simulink model "SF015A_WhlImbRejctn"  (R2013b)
settings: Solver=FixedStepDiscrete  SolverMode=SingleTasking  StartTime=0.0  StopTime=1  FixedStep=0.002  RelTol=1e-3
undefined symbols (not defined in the file): ACTIVBANDMAX_ULS_U32, ADAPVFILMAX_ULS_F32, ADJOUTPMAX_ULS_F32, ARCHGLBPRM_180OVERPI_ULS_F32, ARCHGLBPRM_2MILLISEC_SEC_F32, ARCHGLBPRM_2PI_ULS_F32, ARCHGLBPRM_FLOATZEROTHD_ULS_F32, ARCHGLBPRM_PI_ULS_F32, ARCHGLBPRM_PIOVER180_ULS_F32, ARCHGLBPRM_PIOVER2_ULS_F32, CALMINSPERCOUNT_ULS_F32, Cntr, DURATIONDISABLE_CNT_U16, FILTWHLSPDMAX_MOTRADPERSEC_F32, FRQMIN_ULS_F32, MICROSECTOMILLISEC_ULS_F32, MINSTOMILLISEC_ULS_F32, NINETY_ULS_F32, NODEBSTEP_CNT_U16, NROFDLY_CNT_U08, NtcSts1, NvmGetErrSts1, ONEHALF_ULS_F32, ONEHUNDRED_ULS_F32, ONEOVRTHREE_ULS_F32, ONEOVRTWENTY_ULS_F32, ONETHOUSAND_ULS_F32, PEAKMAX_ULS_F32, PEAKMIN_ULS_F32, PHAADJMAX_ULS_F32, PITIMESSAMPLETIME_ULS_F32, SigQlfr1, STOREDMINSPERCOUNT_ULS_F32, Sts, SysSt1, TWO_ULS_F32, TWOOVRTHREE_ULS_F32, UGRFILMAX_ULS_F32, WhlImbRejctnAdpvFac, WhlImbRejctnAutScaEna, WhlImbRejctnAutScaTar, WhlImbRejctnCurrMgnSlewPerLoop, WhlImbRejctnDcTrendFltRcvryDly, WhlImbRejctnDcTrendFltRcvryNegStep, WhlImbRejctnDcTrendFltRcvryPosStep, WhlImbRejctnDcTrendFltRcvryThd, WhlImbRejctnDcTrendTh2Tq, WhlImbRejctnDcTrendThTq, WhlImbRejctnDcTrendTi2Sec, WhlImbRejctnDcTrendTiSec, WhlImbRejctnEnaSlewPerLoop, WhlImbRejctnFctEna, WhlImbRejctnFltNtc, WhlImbRejctnFrqDiagcAmpThd, WhlImbRejctnFrqDiagcEna, WhlImbRejctnFrqDiagcFltRcvryDly, WhlImbRejctnFrqDiagcFltRcvryNegStep, WhlImbRejctnFrqDiagcFltRcvryPosStep, WhlImbRejctnFrqDiagcFltRcvryThd, WhlImbRejctnFrqDiagcThd ... (+30)
libraries: FixdToFloat x32, simulink x26, NxtrLim x25, Fil x20, NxtrAbslt x9, NxtrMath x7, NxtrMax x6, NxtrMin x4, NxtrNvM x2, FloatToFixd x2, LnrIntrpn x2, NxtrSign x1
(part 3 of 14)

== system SF015A_WhlImbRejctn/WhlImbRejctn/WhlImbRejctnPer1/Active Rejection Command /Adaptive Filter - FloatingL ==
  note: Summation of
      | tapped delay elements
  Enable : Inport
  PrevEpsilon : Inport  Port=2
  AdaptiveMu : Inport  Port=3
  x Ref : Inport  Port=4
  Constant2 : Constant  Value=2  OutDataTypeStr=uint16
  Constant4 : Constant  Value=ADAPVFILMAX_ULS_F32
  CopyRight2 : Subsystem  Description=|  mask(Copyright Information){none=on}
      | Copyright info block.                                               
      |                                                                     
      | Place copyright information at the top of every subsystem in design.
      mask prompts: none "No parameters"
      mask help: Place copyright information at the top of every subsystem in design.
      mask Display:
      | NxtrConf = 'Nexteer Confidential';
      | 
      | sys = bdroot; %handle for the current model ("system")
      | first = get_param(sys,'Created');
      | if(isempty(first))
      |     first = datestr(now,'yyyy');
      | else
      |     first = first(end-3:end);  %year is last four digits
      | end
      | 
      | last = get_param(sys,'LastModifiedDate');
      | if isempty(last)
      |     last = datestr(now,'yyyy');
      | else
      |     last = last(end-3:end);
      | end
      | 
      | if strcmp(first,last)
      |     fprintf('%s -- Copyright %s Nexteer',NxtrConf,first)
      | else
      |     fprintf('%s -- %s%s- %s Nexteer',NxtrConf,char(169),first,last)
      | end
  Data Store Read1 : DataStoreRead  Priority=1  DataStoreName=LeStDlyUpd
      settings: AttributesFormatString=%<Priority>
  Data Store Read2 : DataStoreRead  Priority=1  DataStoreName=LeStVariUpd
      settings: AttributesFormatString=%<Priority>
  Data Store Write1 : DataStoreWrite  Priority=2  DataStoreName=LeStDlyUpd
      settings: AttributesFormatString=%<Priority>
  Data Store Write2 : DataStoreWrite  Priority=3  DataStoreName=LeStVariUpd
      settings: AttributesFormatString=%<Priority>
  Data Store Write3 : DataStoreWrite  DataStoreName=dWhlImbRejctnLMSqdOutLe
  LimDyn_f32 : NxtrLim/LimDyn_f32
  Product3 : Product  RndMeth=Nearest
  Product5 : Product  Inputs=3
  Product6 : Product  RndMeth=Nearest
  Product7 : Product
  Sum3 : Sum  Inputs=|++
  Sum4 : Sum  Inputs=+
  Unary Minus : UnaryMinus
  output : Outport
  wires:
  x Ref/1 -> Data Store Write1/1, Product7/2  "x_k"
  Product3/1 -> Product6/1  "Multiplier"
  [enable] -> Product3/1
  Data Store Read1/1 -> Product6/2  "x_k-1"
  Product7/1 -> Sum4/1
  Product6/1 -> Sum3/1
  Product5/1 -> Product3/2
  AdaptiveMu/1 -> Product5/2
  PrevEpsilon/1 -> Product5/3  "eps_k-1"
  Constant2/1 -> Product5/1
  Enable/1 -> [enable]
  LimDyn_f32/1 -> output/1, Data Store Write3/1
  Data Store Read2/1 -> Sum3/2  "x_k-1"
  Sum3/1 -> Product7/1, Data Store Write2/1
  Sum4/1 -> LimDyn_f32/1  "W_k- xRefStaeVar"
  Constant4/1 -> Unary Minus/1, LimDyn_f32/3
  Unary Minus/1 -> LimDyn_f32/2

== system SF015A_WhlImbRejctn/WhlImbRejctn/WhlImbRejctnPer1/Active Rejection Command /Adaptive Filter - FloatingR ==
  Enable : Inport
  PrevEpsilon : Inport  Port=2
  AdaptiveMu : Inport  Port=3
  x Ref : Inport  Port=4
  Constant1 : Constant  Value=ADAPVFILMAX_ULS_F32
  Constant2 : Constant  Value=2  OutDataTypeStr=uint16
  CopyRight2 : Subsystem  Description=|  mask(Copyright Information){none=on}
      | Copyright info block.                                               
      |                                                                     
      | Place copyright information at the top of every subsystem in design.
      mask prompts: none "No parameters"
      mask help: Place copyright information at the top of every subsystem in design.
      mask Display:
      | NxtrConf = 'Nexteer Confidential';
      | 
      | sys = bdroot; %handle for the current model ("system")
      | first = get_param(sys,'Created');
      | if(isempty(first))
      |     first = datestr(now,'yyyy');
      | else
      |     first = first(end-3:end);  %year is last four digits
      | end
      | 
      | last = get_param(sys,'LastModifiedDate');
      | if isempty(last)
      |     last = datestr(now,'yyyy');
      | else
      |     last = last(end-3:end);
      | end
      | 
      | if strcmp(first,last)
      |     fprintf('%s -- Copyright %s Nexteer',NxtrConf,first)
      | else
      |     fprintf('%s -- %s%s- %s Nexteer',NxtrConf,char(169),first,last)
      | end
  Data Store Read : DataStoreRead  DataStoreName=RiStVariUpd
  Data Store Read1 : DataStoreRead  DataStoreName=RiStDlyUpd
  Data Store Write : DataStoreWrite  DataStoreName=RiStVariUpd
  Data Store Write1 : DataStoreWrite  DataStoreName=RiStDlyUpd
  Data Store Write3 : DataStoreWrite  DataStoreName=dWhlImbRejctnLMSqdOutRi
  LimDyn_f1 : NxtrLim/LimDyn_f32
  Product3 : Product  RndMeth=Nearest
  Product5 : Product  Inputs=3
  Product6 : Product  RndMeth=Nearest
  Product7 : Product
  Sum3 : Sum  Inputs=|++
  Sum4 : Sum  Inputs=+
  Unary Minus1 : UnaryMinus
  output : Outport
  wires:
  Enable/1 -> [enable]
  Constant2/1 -> Product5/1
  PrevEpsilon/1 -> Product5/3  "eps_k-1"
  AdaptiveMu/1 -> Product5/2
  Product5/1 -> Product3/2
  Product6/1 -> Sum3/1
  Product7/1 -> Sum4/1
  [enable] -> Product3/1
  Product3/1 -> Product6/1  "Multiplier"
  x Ref/1 -> Data Store Write1/1, Product7/2  "x_k"
  Data Store Read1/1 -> Product6/2  "x_k-1"
  Data Store Read/1 -> Sum3/2  "x_k-1"
  LimDyn_f1/1 -> Data Store Write3/1, output/1
  Sum3/1 -> Product7/1, Data Store Write/1
  Sum4/1 -> LimDyn_f1/1  "W_k- xRefStaeVar"
  Constant1/1 -> Unary Minus1/1, LimDyn_f1/3
  Unary Minus1/1 -> LimDyn_f1/2

== system SF015A_WhlImbRejctn/WhlImbRejctn/WhlImbRejctnPer1/Active Rejection Command /Amplitude Calculation ==
  Input : Inport
  Abslt_f32_f32 : NxtrAbslt/Abslt_f32_f32  SFunctionSpec=single y1 = Abslt_f32_f32(single u1)
      settings: AttributesFormatString=%<Name>
  Constant : Constant  Value=ARCHGLBPRM_PIOVER2_ULS_F32
  CopyRight2 : Subsystem  Description=|  mask(Copyright Information){none=on}
      | Copyright info block.                                               
      |                                                                     
      | Place copyright information at the top of every subsystem in design.
      mask prompts: none "No parameters"
      mask help: Place copyright information at the top of every subsystem in design.
      mask Display:
      | NxtrConf = 'Nexteer Confidential';
      | 
      | sys = bdroot; %handle for the current model ("system")
      | first = get_param(sys,'Created');
      | if(isempty(first))
      |     first = datestr(now,'yyyy');
      | else
      |     first = first(end-3:end);  %year is last four digits
      | end
      | 
      | last = get_param(sys,'LastModifiedDate');
      | if isempty(last)
      |     last = datestr(now,'yyyy');
      | else
      |     last = last(end-3:end);
      | end
      | 
      | if strcmp(first,last)
      |     fprintf('%s -- Copyright %s Nexteer',NxtrConf,first)
      | else
      |     fprintf('%s -- %s%s- %s Nexteer',NxtrConf,char(169),first,last)
      | end
  FilLpUpdOutp : Fil/FilLpUpdOutp  StVar=CmdMgnLp1Fil
      settings: AttributesFormatString=StVar: %<StVar>
  FilLpUpdOutp1 : Fil/FilLpUpdOutp  StVar=CmdMgnLp2Fil
      settings: AttributesFormatString=StVar: %<StVar>
  Product : Product
  Amp : Outport
  wires:
  FilLpUpdOutp1/1 -> Amp/1
  Abslt_f32_f32/1 -> FilLpUpdOutp/1
  Product/1 -> FilLpUpdOutp1/1
  FilLpUpdOutp/1 -> Product/1
  Input/1 -> Abslt_f32_f32/1
  Constant/1 -> Product/2

== system SF015A_WhlImbRejctn/WhlImbRejctn/WhlImbRejctnPer1/Active Rejection Command /CopyRight2 ==

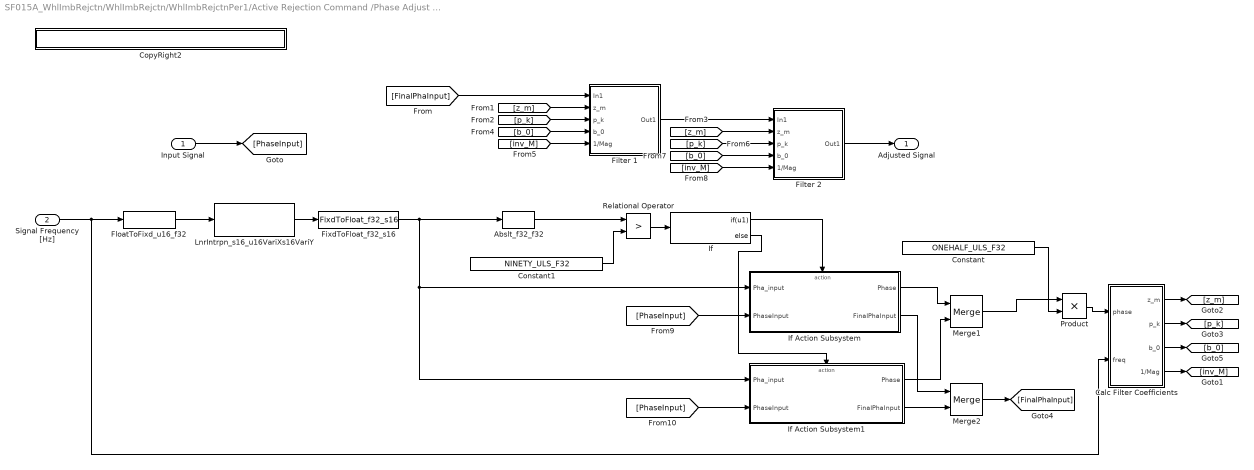
== system SF015A_WhlImbRejctn/WhlImbRejctn/WhlImbRejctnPer1/Active Rejection Command /Phase Adjust - Floating Point ==
  Input Signal : Inport
  Signal Frequency [Hz] : Inport  Port=2
  Abslt_f32_f32 : NxtrAbslt/Abslt_f32_f32  SFunctionSpec=single y1 = Abslt_f32_f32(single u1)
      settings: AttributesFormatString=%<Name>
  Calc Filter Coefficients : Subsystem
  Constant : Constant  Value=ONEHALF_ULS_F32
  Constant1 : Constant  Value=NINETY_ULS_F32
  CopyRight2 : Subsystem  Description=|  mask(Copyright Information){none=on}
      | Copyright info block.                                               
      |                                                                     
      | Place copyright information at the top of every subsystem in design.
      mask prompts: none "No parameters"
      mask help: Place copyright information at the top of every subsystem in design.
      mask Display:
      | NxtrConf = 'Nexteer Confidential';
      | 
      | sys = bdroot; %handle for the current model ("system")
      | first = get_param(sys,'Created');
      | if(isempty(first))
      |     first = datestr(now,'yyyy');
      | else
      |     first = first(end-3:end);  %year is last four digits
      | end
      | 
      | last = get_param(sys,'LastModifiedDate');
      | if isempty(last)
      |     last = datestr(now,'yyyy');
      | else
      |     last = last(end-3:end);
      | end
      | 
      | if strcmp(first,last)
      |     fprintf('%s -- Copyright %s Nexteer',NxtrConf,first)
      | else
      |     fprintf('%s -- %s%s- %s Nexteer',NxtrConf,char(169),first,last)
      | end
  Filter 1 : Subsystem
  Filter 2 : Subsystem
  FixdToFloat_f32_s16 : FixdToFloat/FixdToFloat_f32_s16  Param1=7
  FloatToFixd_u16_f32 : FloatToFixd/FloatToFixd_u16_f32  Param1=9
  If : If  IfExpression=u1
  If Action Subsystem : Subsystem  TreatAsAtomicUnit=on
  If Action Subsystem1 : Subsystem  TreatAsAtomicUnit=on
  LnrIntrpn_s16_u16VariXs16VariY : LnrIntrpn/LnrIntrpn_s16_u16VariXs16VariY  XTbl=WhlImbRejctnPhaAdjX  YTbl=WhlImbRejctnPhaAdjY
      settings: AttributesFormatString=Lnr ( u16VariX , s16VariY )
  Merge1 : Merge
  Merge2 : Merge
  Product : Product
  Relational Operator : RelationalOperator  Operator=>  OutDataTypeStr=boolean
  Adjusted Signal : Outport
  wires:
  Filter 2/1(Out1) -> Adjusted Signal/1
  Filter 1/1(Out1) -> Filter 2/1(In1)
  [inv_M] -> Filter 2/5(1/Mag)
  [b_0] -> Filter 2/4(b_0)
  [p_k] -> Filter 2/3(p_k)
  [z_m] -> Filter 2/2(z_m)
  [inv_M] -> Filter 1/5(1/Mag)
  [b_0] -> Filter 1/4(b_0)
  [p_k] -> Filter 1/3(p_k)
  [z_m] -> Filter 1/2(z_m)
  Calc Filter Coefficients/4(1/Mag) -> [inv_M]
  Calc Filter Coefficients/2(p_k) -> [p_k]
  Calc Filter Coefficients/1(z_m) -> [z_m]
  Calc Filter Coefficients/3(b_0) -> [b_0]
  FixdToFloat_f32_s16/1 -> If Action Subsystem1/1(Pha_input), If Action Subsystem/1(Pha_input), Abslt_f32_f32/1
  Input Signal/1 -> [PhaseInput]
  FloatToFixd_u16_f32/1 -> LnrIntrpn_s16_u16VariXs16VariY/1
  Relational Operator/1 -> If/1
  If/1 -> If Action Subsystem/Action
  [PhaseInput] -> If Action Subsystem/2(PhaseInput)
  Merge2/1 -> [FinalPhaInput]
  Merge1/1 -> Product/1
  If/2 -> If Action Subsystem1/Action
  [PhaseInput] -> If Action Subsystem1/2(PhaseInput)
  If Action Subsystem/1(Phase) -> Merge1/1
  If Action Subsystem1/1(Phase) -> Merge1/2
  If Action Subsystem/2(FinalPhaInput) -> Merge2/1
  If Action Subsystem1/2(FinalPhaInput) -> Merge2/2
  Signal Frequency [Hz]/1 -> Calc Filter Coefficients/2(freq), FloatToFixd_u16_f32/1
  [FinalPhaInput] -> Filter 1/1(In1)
  Product/1 -> Calc Filter Coefficients/1(phase)
  Constant/1 -> Product/2
  Abslt_f32_f32/1 -> Relational Operator/1
  Constant1/1 -> Relational Operator/2
  LnrIntrpn_s16_u16VariXs16VariY/1 -> FixdToFloat_f32_s16/1

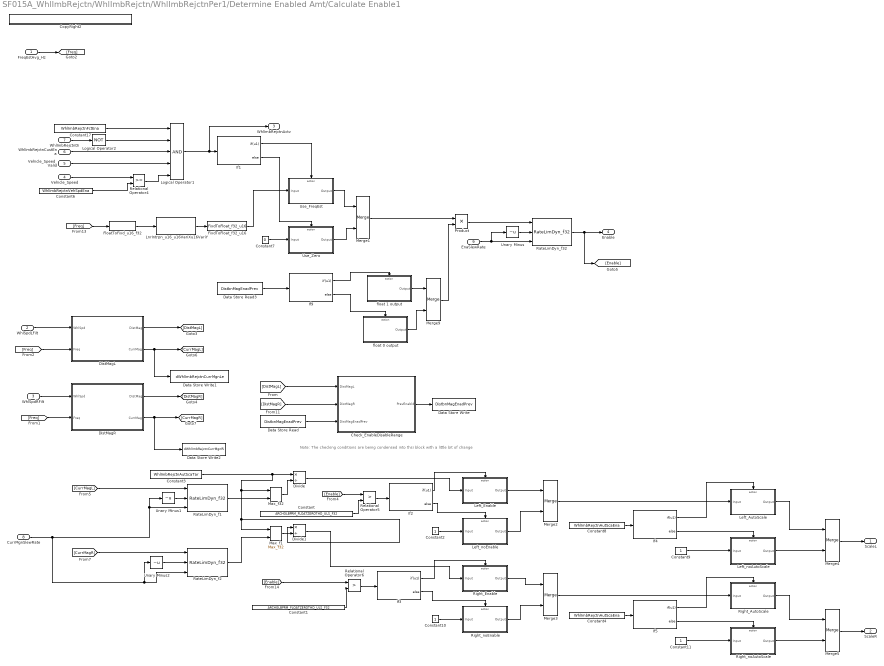
== system SF015A_WhlImbRejctn/WhlImbRejctn/WhlImbRejctnPer1/Determine Enabled Amt/Calculate Enable1 ==
  note: Note: The checking conditions are being condensed into thsi block with a little bit of change
  FreqEstAvg_Hz : Inport
  WhlSpdLFilt : Inport  Port=2
  WhlSpdRFilt : Inport  Port=3
  Vehicle_Speed : Inport  Port=4
  Vehicle_Speed_Valid : Inport  Port=5
  WhlImbRejctnCustEna : Inport  Port=6
  WhlImbRejctnDi : Inport  Port=7
  CurrMgnSlewRate : Inport  Port=8
  EnaSlewRate : Inport  Port=9
  Check_EnableDisableRange : Subsystem
  Constant : Constant  Value=ARCHGLBPRM_FLOATZEROTHD_ULS_F32
  Constant1 : Constant  Value=ARCHGLBPRM_FLOATZEROTHD_ULS_F32
  Constant{2,9..11} (4 alike) : Constant  OutDataTypeStr=single
  Constant17 : Constant  Value=WhlImbRejctnFctEna
  Constant3 : Constant  Value=WhlImbRejctnAutScaTar
  Constant4 : Constant  Value=WhlImbRejctnAutScaEna
  Constant6 : Constant  Value=WhlImbRejctnVehSpdEna
  Constant7 : Constant  Value=0  OutDataTypeStr=single
  Constant8 : Constant  Value=WhlImbRejctnAutScaEna
  CopyRight2 : Subsystem  Description=|  mask(Copyright Information){none=on}
      | Copyright info block.                                               
      |                                                                     
      | Place copyright information at the top of every subsystem in design.
      mask prompts: none "No parameters"
      mask help: Place copyright information at the top of every subsystem in design.
      mask Display:
      | NxtrConf = 'Nexteer Confidential';
      | 
      | sys = bdroot; %handle for the current model ("system")
      | first = get_param(sys,'Created');
      | first = first(end-3:end);  %year is last four digits
      | 
      | last = get_param(sys,'LastModifiedDate');
      | if isempty(last)
      |     last = datestr(now,'yyyy');
      | else
      |     last = last(end-3:end);
      | end
      | 
      | if strcmp(first,last)
      |     fprintf('%s -- Copyright %s Nexteer',NxtrConf,first)
      | else
      |     fprintf('%s -- %s%s- %s Nexteer',NxtrConf,char(169),first,last)
      | end
  Data Store Read : DataStoreRead  Priority=2  DataStoreName=DistbnMagEnadPrev
      settings: AttributesFormatString=Priority=%<Priority>
  Data Store Read3 : DataStoreRead  Priority=1  DataStoreName=DistbnMagEnadPrev
      settings: AttributesFormatString=Priority=%<Priority>
  Data Store Write : DataStoreWrite  Priority=3  DataStoreName=DistbnMagEnadPrev
      settings: AttributesFormatString=Priority=%<Priority>
  Data Store Write1 : DataStoreWrite  DataStoreName=dWhlImbRejctnCurrMgnLe
  Data Store Write2 : DataStoreWrite  DataStoreName=dWhlImbRejctnCurrMgnRi
  DistMagL : Subsystem
  DistMagR : Subsystem
  Divide : Product  Inputs=*/
  Divide1 : Product  Inputs=*/
  FixdToFloat_f32_u16 : FixdToFloat/FixdToFloat_f32_u16  Param1=15
  FloatToFixd_u16_f32 : FloatToFixd/FloatToFixd_u16_f32  Param1=10
  If1 : If  RequirementInfo={} %GIDa_7d8297b8_b265_4b47_b8b2_192e5a92e4fb  IfExpression=u1
  If2 : If  RequirementInfo={} %GIDa_0556d171_7866_4516_8d40_956f321be7bc  IfExpression=u1
  If3 : If  RequirementInfo={} %GIDa_fcbce161_0599_4b7a_b23c_d7b8d7e27a0f  IfExpression=u1
  If4 : If  RequirementInfo={} %GIDa_46a5a10e_d4b7_40a4_ac58_d797cb624c83  IfExpression=u1
  If5 : If  RequirementInfo={} %GIDa_3e7d8d50_75ba_4493_bb61_e3ba5f1e5c7c  IfExpression=u1
  If9 : If  RequirementInfo={} %GIDa_220c56c6_5b09_48da_a4b3_63431d3edf67  IfExpression=u1
  Left_AutoScale : Subsystem  RequirementInfo={} %GIDa_9c3ac42f_cbc1_49be_98f6_7ec1737ed2ed  TreatAsAtomicUnit=on
  Left_Enable : Subsystem  RequirementInfo={} %GIDa_d65479b8_5b54_4e68_bf36_3b31ad24537e  TreatAsAtomicUnit=on
  Left_noAutoScale : Subsystem  RequirementInfo={} %GIDa_bdc4660b_a72c_40f0_89ba_28a8acc1db11  TreatAsAtomicUnit=on
  Left_noEnable : Subsystem  RequirementInfo={} %GIDa_18e28b2f_1f1d_4076_8343_147cb5570336  TreatAsAtomicUnit=on
  LnrIntrpn_u16_u16VariXu16VariY : LnrIntrpn/LnrIntrpn_u16_u16VariXu16VariY  XTbl=WhlImbRejctnFrqScaTblX  YTbl=WhlImbRejctnFrqScaTblY
      settings: AttributesFormatString=Lnr ( u16VariX , u16VariY )
  Logical Operator1 : Logic  Inputs=5  AllPortsSameDT=off  OutDataTypeStr=boolean
  Logical Operator2 : Logic  Operator=NOT  Inputs=5  AllPortsSameDT=off  OutDataTypeStr=boolean
  Max_f1 : NxtrMax/Max_f32  SFunctionSpec=single y1 = Max_f32(single u1, single u2)
      settings: AttributesFormatString=%<Name>
  Max_f32 : NxtrMax/Max_f32  SFunctionSpec=single y1 = Max_f32(single u1, single u2)
      settings: AttributesFormatString=%<Name>
  Merge{1..5,9} (6 alike) : Merge
  Product : Product
  RateLimDyn_f1 : NxtrLim/RateLimDyn_f32  StVar=LeCurrMgnSlewPerLoop  Ts=ARCHGLBPRM_2MILLISEC_SEC_F32
      settings: AttributesFormatString=StVar: %<StVar>
  RateLimDyn_f2 : NxtrLim/RateLimDyn_f32  StVar=RiCurrMgnSlewPerLoop  Ts=ARCHGLBPRM_2MILLISEC_SEC_F32
      settings: AttributesFormatString=StVar: %<StVar>
  RateLimDyn_f32 : NxtrLim/RateLimDyn_f32  StVar=EnaSlewPerLoop  Ts=ARCHGLBPRM_2MILLISEC_SEC_F32
      settings: AttributesFormatString=StVar: %<StVar>
  Relational Operator4 : RelationalOperator  OutDataTypeStr=boolean
  Relational Operator5 : RelationalOperator  Operator=>  OutDataTypeStr=boolean
  Relational Operator6 : RelationalOperator  Operator=>  OutDataTypeStr=boolean
  Right_AutoScale : Subsystem  RequirementInfo={} %GIDa_13da9aa5_5c49_428f_b287_6188729282ed  TreatAsAtomicUnit=on
  Right_Enable : Subsystem  RequirementInfo={} %GIDa_75bbbddb_2767_47a3_9165_63797ed0e216  TreatAsAtomicUnit=on
  Right_noAutoScale : Subsystem  RequirementInfo={} %GIDa_e3eec680_517e_4da7_948a_b3f8124b2971  TreatAsAtomicUnit=on
  Right_noEnable : Subsystem  RequirementInfo={} %GIDa_b2607bc0_d58b_406c_8b11_3dee4f11cd4c  TreatAsAtomicUnit=on
  Unary Minus : UnaryMinus
  Unary Minus1 : UnaryMinus
  Unary Minus2 : UnaryMinus
  Use_FreqEst : Subsystem  RequirementInfo={} %GIDa_066b3e73_a3fa_4d6c_9937_967fb698f328  TreatAsAtomicUnit=on
  Use_Zero : Subsystem  RequirementInfo={} %GIDa_7b829dcd_761e_44e8_86d6_74abc0632468  TreatAsAtomicUnit=on
  float 0 output : Subsystem  RequirementInfo={} %GIDa_73b9442c_5069_415a_a71a_08570183037e  TreatAsAtomicUnit=on
  float 1 output : Subsystem  RequirementInfo={} %GIDa_eb48623e_e509_47ed_bd29_5bcb251c6a65  TreatAsAtomicUnit=on
  ScaleL : Outport
  ScaleR : Outport  Port=2
  WhlImbRejctnActv : Outport  Port=3
  Enable : Outport  Port=4
  wires:
  FreqEstAvg_Hz/1 -> [Freq]
  WhlSpdLFilt/1 -> DistMagL/1(WhlSpd)
  [Freq] -> DistMagL/2(Freq)
  WhlSpdRFilt/1 -> DistMagR/1(WhlSpd)
  [Freq] -> DistMagR/2(Freq)
  DistMagL/1(DistMag) -> [DistMagL]
  DistMagR/1(DistMag) -> [DistMagR]
  Data Store Read3/1 -> If9/1
  Constant3/1 -> Max_f32/1, Max_f1/1, Divide1/1, Divide/1
  DistMagL/2(CurrMag) -> Data Store Write1/1, [CurrMagL]
  DistMagR/2(CurrMag) -> Data Store Write2/1, [CurrMagR]
  Max_f32/1 -> Divide/2
  [CurrMagL] -> RateLimDyn_f1/1
  Max_f1/1 -> Divide1/2
  [CurrMagR] -> RateLimDyn_f2/1
  Vehicle_Speed/1 -> Relational Operator4/1
  Constant6/1 -> Relational Operator4/2
  Relational Operator4/1 -> Logical Operator1/5
  Vehicle_Speed_Valid/1 -> Logical Operator1/4
  WhlImbRejctnCustEna/1 -> Logical Operator1/3
  WhlImbRejctnDi/1 -> Logical Operator2/1
  Constant7/1 -> Use_Zero/1(Input)
  If1/1 -> Use_FreqEst/Action
  If1/2 -> Use_Zero/Action
  Logical Operator1/1 -> WhlImbRejctnActv/1, If1/1
  Use_FreqEst/1(Output) -> Merge1/1
  Use_Zero/1(Output) -> Merge1/2
  Merge1/1 -> Product/1
  [Freq] -> FloatToFixd_u16_f32/1
  FixdToFloat_f32_u16/1 -> Use_FreqEst/1(Input)
  LnrIntrpn_u16_u16VariXu16VariY/1 -> FixdToFloat_f32_u16/1
  FloatToFixd_u16_f32/1 -> LnrIntrpn_u16_u16VariXu16VariY/1
  Product/1 -> RateLimDyn_f32/1
  Constant2/1 -> Left_noEnable/1(Input)
  If2/1 -> Left_Enable/Action
  If2/2 -> Left_noEnable/Action
  Left_Enable/1(Output) -> Merge2/1
  Left_noEnable/1(Output) -> Merge2/2
  Divide/1 -> Left_Enable/1(Input)
  [Enable] -> Relational Operator5/1
  Constant10/1 -> Right_noEnable/1(Input)
  If3/1 -> Right_Enable/Action
  If3/2 -> Right_noEnable/Action
  Right_Enable/1(Output) -> Merge3/1
  Right_noEnable/1(Output) -> Merge3/2
  Divide1/1 -> Right_Enable/1(Input)
  If4/1 -> Left_AutoScale/Action
  If4/2 -> Left_noAutoScale/Action
  Left_AutoScale/1(Output) -> Merge4/1
  Left_noAutoScale/1(Output) -> Merge4/2
  Merge2/1 -> Left_AutoScale/1(Input)
  Constant8/1 -> If4/1
  Merge4/1 -> ScaleL/1
  Constant9/1 -> Left_noAutoScale/1(Input)
  If5/1 -> Right_AutoScale/Action
  If5/2 -> Right_noAutoScale/Action
  Right_AutoScale/1(Output) -> Merge5/1
  Right_noAutoScale/1(Output) -> Merge5/2
  Merge3/1 -> Right_AutoScale/1(Input)
  Constant4/1 -> If5/1
  Constant11/1 -> Right_noAutoScale/1(Input)
  Merge5/1 -> ScaleR/1
  RateLimDyn_f32/1 -> Enable/1, [Enable]
  Unary Minus/1 -> RateLimDyn_f32/2
  Unary Minus1/1 -> RateLimDyn_f1/2
  RateLimDyn_f1/1 -> Max_f32/2
  CurrMgnSlewRate/1 -> RateLimDyn_f2/3, Unary Minus2/1, Unary Minus1/1, RateLimDyn_f1/3
  Unary Minus2/1 -> RateLimDyn_f2/2
  RateLimDyn_f2/1 -> Max_f1/2
  Constant17/1 -> Logical Operator1/1
  Merge9/1 -> Product/2
  Relational Operator5/1 -> If2/1
  Relational Operator6/1 -> If3/1
  EnaSlewRate/1 -> Unary Minus/1, RateLimDyn_f32/3
  Constant/1 -> Relational Operator5/2
  [Enable] -> Relational Operator6/1
  Constant1/1 -> Relational Operator6/2
  If9/1 -> float 1 output/Action
  float 1 output/1(Output) -> Merge9/1
  If9/2 -> float 0 output/Action
  float 0 output/1(Output) -> Merge9/2
  Logical Operator2/1 -> Logical Operator1/2
  [DistMagL] -> Check_EnableDisableRange/1(DistMagL)
  [DistMagR] -> Check_EnableDisableRange/2(DistMagR)
  Data Store Read/1 -> Check_EnableDisableRange/3(DistMagEnadPrev)
  Check_EnableDisableRange/1(PrevEnabld) -> Data Store Write/1

== system SF015A_WhlImbRejctn/WhlImbRejctn/WhlImbRejctnPer1/Determine Enabled Amt/CopyRight2 ==

== system SF015A_WhlImbRejctn/WhlImbRejctn/WhlImbRejctnPer1/Determine Enabled Amt/Enable Ramp ==
  Enable In : Inport
  "RampY " : Inport  Port=2
  RampN : Inport  Port=3
  SYSTEM_STATE : Inport  Port=4
  Constant : Constant  Value=0  OutDataTypeStr=single
  Constant6 : Constant  Value=ARCHGLBPRM_FLOATZEROTHD_ULS_F32
  CopyRight2 : Subsystem  Description=|  mask(Copyright Information){none=on}
      | Copyright info block.                                               
      |                                                                     
      | Place copyright information at the top of every subsystem in design.
      mask prompts: none "No parameters"
      mask help: Place copyright information at the top of every subsystem in design.
      mask Display:
      | NxtrConf = 'Nexteer Confidential';
      | 
      | sys = bdroot; %handle for the current model ("system")
      | first = get_param(sys,'Created');
      | first = first(end-3:end);  %year is last four digits
      | 
      | last = get_param(sys,'LastModifiedDate');
      | if isempty(last)
      |     last = datestr(now,'yyyy');
      | else
      |     last = last(end-3:end);
      | end
      | 
      | if strcmp(first,last)
      |     fprintf('%s -- Copyright %s Nexteer',NxtrConf,first)
      | else
      |     fprintf('%s -- %s%s- %s Nexteer',NxtrConf,char(169),first,last)
      | end
  ElapsedTime1 : Subsystem  TreatAsAtomicUnit=on
  Enumerated Constant : simulink/Sources/Enumerated Constant  OutDataTypeStr=Enum: SysSt1  Value=SysSt1.SYSST_ENA  SampleTime=inf
  If1 : If  RequirementInfo={} %GIDa_bfd6920b_006a_416f_b6f7_6ef0775419c8  IfExpression=u1
  If2 : If  RequirementInfo={} %GIDa_894989e0_ef65_43c4_bfdb_f22d51c8efad  IfExpression=u1  ShowElse=off
  If7 : If  RequirementInfo={} %GIDa_516cf2d0_a63b_46fe_b255_3d41307786bb  IfExpression=u1
  Logical Operator1 : Logic  AllPortsSameDT=off  OutDataTypeStr=boolean
  Logical Operator2 : Logic  Operator=OR  AllPortsSameDT=off  OutDataTypeStr=boolean
  Logical Operator4 : Logic  AllPortsSameDT=off  OutDataTypeStr=boolean
  Merge1 : Merge
  Merge7 : Merge
  NoFaultOper : Subsystem  RequirementInfo={} %GIDa_85bb45c8_b5a9_4bce_b96d_1bcc95564bc7  TreatAsAtomicUnit=on
  Relational Operator1 : RelationalOperator  Operator===  OutDataTypeStr=boolean
  Relational Operator9 : RelationalOperator  Operator=<=  OutDataTypeStr=boolean
  "Reset WIR " : Subsystem  TreatAsAtomicUnit=on
  Right_active1 : Subsystem  RequirementInfo={} %GIDa_d211d460_285e_47ce_a10a_276eb1a21d5a  TreatAsAtomicUnit=on
  Right_noactive1 : Subsystem  RequirementInfo={} %GIDa_3ffdf98d_b314_4708_8422_325b4c42ba1c  TreatAsAtomicUnit=on
  SlowSpeedDiagcCalc : Subsystem  RequirementInfo={} %GIDa_b7c7be65_73bf_45a8_bfe0_fa96a024938d  TreatAsAtomicUnit=on
  Ramped Enable : Outport
  wires:
  Constant6/1 -> Relational Operator9/2
  Relational Operator9/1 -> Logical Operator4/1
  Logical Operator4/1 -> Logical Operator2/2
  Logical Operator1/1 -> If2/1
  Enable In/1 -> [Enable_In]
  "RampY "/1 -> [RampY]
  [RampN] -> Logical Operator2/1
  If7/1 -> SlowSpeedDiagcCalc/Action
  If7/2 -> NoFaultOper/Action
  NoFaultOper/1(Output) -> Merge7/2
  [Enable_In] -> NoFaultOper/1(Input)
  If1/1 -> Right_active1/Action
  If1/2 -> Right_noactive1/Action
  Right_active1/1(Output) -> Merge1/1
  Right_noactive1/1(Output) -> Merge1/2
  Merge7/1 -> Right_noactive1/1(Input)  "RampDwnScaleFactor"
  Constant/1 -> Right_active1/1(Input)
  [RampN] -> If1/1
  Merge1/1 -> Ramped Enable/1
  [Enable_In] -> SlowSpeedDiagcCalc/1(EnableScaleFactor)
  RampN/1 -> [RampN]
  [RampY] -> Logical Operator4/2
  [RampYElapsdTi] -> SlowSpeedDiagcCalc/2(RampYElapsdTi)
  [RampY] -> If7/1
  If2/1 -> "Reset WIR "/Action
  SYSTEM_STATE/1 -> Relational Operator1/1
  Enumerated Constant/1 -> Relational Operator1/2
  Logical Operator2/1 -> Logical Operator1/1
  Relational Operator1/1 -> Logical Operator1/2
  SlowSpeedDiagcCalc/1(Output) -> Relational Operator9/1
  SlowSpeedDiagcCalc/2(Output1) -> Merge7/1
  [RampY] -> ElapsedTime1/1(FltStsTrue)
  ElapsedTime1/1(ElapsedTime) -> [RampYElapsdTi]

== system SF015A_WhlImbRejctn/WhlImbRejctn/WhlImbRejctnPer1/WIR Diagnostics/Amplitude Calculation1 ==
  Input : Inport
  Abslt_f32_f32 : NxtrAbslt/Abslt_f32_f32  SFunctionSpec=single y1 = Abslt_f32_f32(single u1)
      settings: AttributesFormatString=%<Name>
  Constant : Constant  Value=ARCHGLBPRM_PIOVER2_ULS_F32
  CopyRight2 : Subsystem  Description=|  mask(Copyright Information){none=on}
      | Copyright info block.                                               
      |                                                                     
      | Place copyright information at the top of every subsystem in design.
      mask prompts: none "No parameters"
      mask help: Place copyright information at the top of every subsystem in design.
      mask Display:
      | NxtrConf = 'Nexteer Confidential';
      | 
      | sys = bdroot; %handle for the current model ("system")
      | first = get_param(sys,'Created');
      | first = first(end-3:end);  %year is last four digits
      | 
      | last = get_param(sys,'LastModifiedDate');
      | if isempty(last)
      |     last = datestr(now,'yyyy');
      | else
      |     last = last(end-3:end);
      | end
      | 
      | if strcmp(first,last)
      |     fprintf('%s -- Copyright %s Nexteer',NxtrConf,first)
      | else
      |     fprintf('%s -- %s%s- %s Nexteer',NxtrConf,char(169),first,last)
      | end
  FilLpUpdOutp : Fil/FilLpUpdOutp  StVar=BlndCmdMgnLp1Fil
      settings: AttributesFormatString=StVar: %<StVar>
  FilLpUpdOutp1 : Fil/FilLpUpdOutp  StVar=BlndCmdMgnLp2Fil
      settings: AttributesFormatString=StVar: %<StVar>
  Product : Product
  Amp : Outport
  wires:
  FilLpUpdOutp1/1 -> Amp/1
  FilLpUpdOutp/1 -> Product/1
  Abslt_f32_f32/1 -> FilLpUpdOutp/1
  Input/1 -> Abslt_f32_f32/1
  Product/1 -> FilLpUpdOutp1/1
  Constant/1 -> Product/2

== system SF015A_WhlImbRejctn/WhlImbRejctn/WhlImbRejctnPer1/WIR Diagnostics/CopyRight2 ==

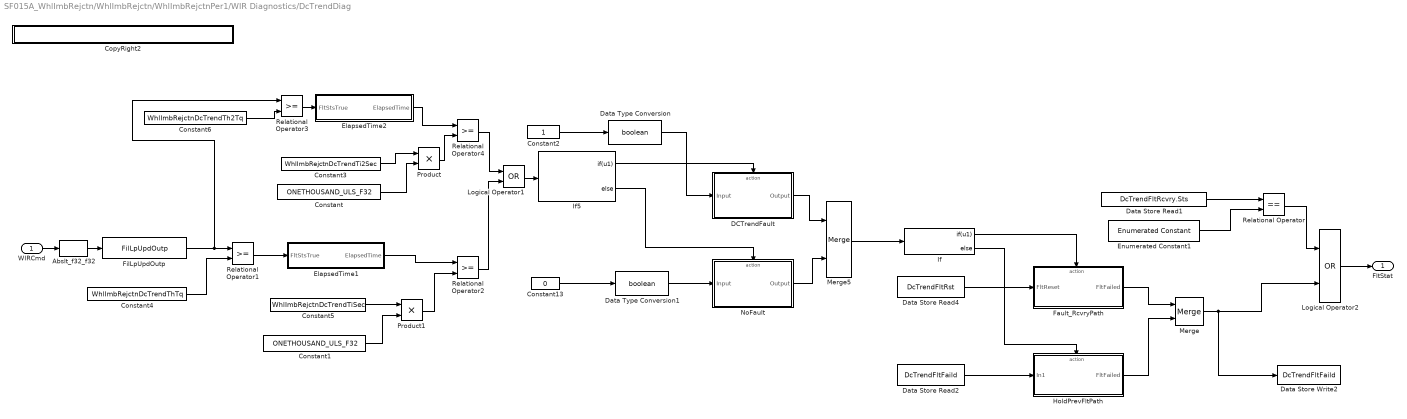
== system SF015A_WhlImbRejctn/WhlImbRejctn/WhlImbRejctnPer1/WIR Diagnostics/DcTrendDiag ==
  WIRCmd : Inport
  Abslt_f32_f32 : NxtrAbslt/Abslt_f32_f32  SFunctionSpec=single y1 = Abslt_f32_f32(single u1)
      settings: AttributesFormatString=%<Name>
  Constant : Constant  Value=ONETHOUSAND_ULS_F32
  Constant1 : Constant  Value=ONETHOUSAND_ULS_F32
  Constant13 : Constant  Value=0  OutDataTypeStr=boolean
  Constant2 : Constant  OutDataTypeStr=Inherit: Inherit via back propagation
  Constant3 : Constant  Value=WhlImbRejctnDcTrendTi2Sec
  Constant4 : Constant  Value=WhlImbRejctnDcTrendThTq
  Constant5 : Constant  Value=WhlImbRejctnDcTrendTiSec
  Constant6 : Constant  Value=WhlImbRejctnDcTrendTh2Tq
  CopyRight2 : Subsystem  Description=|  mask(Copyright Information){none=on}
      | Copyright info block.                                               
      |                                                                     
      | Place copyright information at the top of every subsystem in design.
      mask prompts: none "No parameters"
      mask help: Place copyright information at the top of every subsystem in design.
      mask Display:
      | NxtrConf = 'Nexteer Confidential';
      | 
      | sys = bdroot; %handle for the current model ("system")
      | first = get_param(sys,'Created');
      | first = first(end-3:end);  %year is last four digits
      | 
      | last = get_param(sys,'LastModifiedDate');
      | if isempty(last)
      |     last = datestr(now,'yyyy');
      | else
      |     last = last(end-3:end);
      | end
      | 
      | if strcmp(first,last)
      |     fprintf('%s -- Copyright %s Nexteer',NxtrConf,first)
      | else
      |     fprintf('%s -- %s%s- %s Nexteer',NxtrConf,char(169),first,last)
      | end
  DCTrendFault : Subsystem  RequirementInfo={} %GIDa_a2bf172f_152a_4264_a2d8_48cf318cb81e  TreatAsAtomicUnit=on
  Data Store Read1 : DataStoreRead  DataStoreName=DcTrendFltRcvry  DataStoreElements=DcTrendFltRcvry.Sts
  Data Store Read2 : DataStoreRead  Priority=1  DataStoreName=DcTrendFltFaild
      settings: AttributesFormatString=Priority:%<Priority>
  Data Store Read4 : DataStoreRead  Priority=1  DataStoreName=DcTrendFltRst
      settings: AttributesFormatString=Priority:%<Priority>
  Data Store Write2 : DataStoreWrite  Priority=2  DataStoreName=DcTrendFltFaild
      settings: AttributesFormatString=Priority:%<Priority>
  Data Type Conversion : DataTypeConversion  OutDataTypeStr=boolean
  Data Type Conversion1 : DataTypeConversion  OutDataTypeStr=boolean
  ElapsedTime1 : Subsystem  TreatAsAtomicUnit=on
  ElapsedTime2 : Subsystem  TreatAsAtomicUnit=on
  Enumerated Constant1 : simulink/Sources/Enumerated Constant  OutDataTypeStr=Enum: SigQlfr1  Value=SigQlfr1.SIGQLFR_FAILD  SampleTime=inf
  Fault_RcvryPath : Subsystem  TreatAsAtomicUnit=on
  FilLpUpdOutp : Fil/FilLpUpdOutp  StVar=DcTrendLpFil
      settings: AttributesFormatString=StVar: %<StVar>
  HoldPrevFltPath : Subsystem  TreatAsAtomicUnit=on
  If : If  IfExpression=u1
  If5 : If  RequirementInfo={} %GIDa_0ecf552f_0a22_4e50_8225_2e691f1dcd0f  IfExpression=u1
  Logical Operator1 : Logic  Operator=OR  AllPortsSameDT=off  OutDataTypeStr=boolean
  Logical Operator2 : Logic  Operator=OR  AllPortsSameDT=off  OutDataTypeStr=boolean
  Merge : Merge
  Merge5 : Merge
  NoFault : Subsystem  RequirementInfo={} %GIDa_b91ed932_8d0a_4501_94cd_eecd5662fa49  TreatAsAtomicUnit=on
  Product : Product
  Product1 : Product
  Relational Operator : RelationalOperator  Operator===  OutDataTypeStr=boolean
  Relational Operator{1..4} (4 alike) : RelationalOperator  OutDataTypeStr=boolean
  FltStat : Outport
  wires:
  Abslt_f32_f32/1 -> FilLpUpdOutp/1
  FilLpUpdOutp/1 -> Relational Operator1/1, Relational Operator3/1
  Constant4/1 -> Relational Operator1/2
  Relational Operator1/1 -> ElapsedTime1/1(FltStsTrue)
  ElapsedTime1/1(ElapsedTime) -> Relational Operator2/1
  Relational Operator3/1 -> ElapsedTime2/1(FltStsTrue)
  Constant3/1 -> Product/1
  Constant6/1 -> Relational Operator3/2
  Logical Operator1/1 -> If5/1
  Relational Operator4/1 -> Logical Operator1/1
  Relational Operator2/1 -> Logical Operator1/2
  If5/1 -> DCTrendFault/Action
  If5/2 -> NoFault/Action
  DCTrendFault/1(Output) -> Merge5/1
  NoFault/1(Output) -> Merge5/2
  Constant2/1 -> Data Type Conversion/1
  Constant13/1 -> Data Type Conversion1/1
  WIRCmd/1 -> Abslt_f32_f32/1
  Data Type Conversion/1 -> DCTrendFault/1(Input)
  Data Type Conversion1/1 -> NoFault/1(Input)
  ElapsedTime2/1(ElapsedTime) -> Relational Operator4/1
  Constant/1 -> Product/2
  Product/1 -> Relational Operator4/2
  Constant1/1 -> Product1/2
  Product1/1 -> Relational Operator2/2
  Constant5/1 -> Product1/1
  Merge5/1 -> If/1
  Data Store Read4/1 -> Fault_RcvryPath/1(FltReset)
  If/1 -> Fault_RcvryPath/Action
  Fault_RcvryPath/1(FltFailed) -> Merge/1
  HoldPrevFltPath/1(FltFailed) -> Merge/2
  If/2 -> HoldPrevFltPath/Action
  Enumerated Constant1/1 -> Relational Operator/2
  Relational Operator/1 -> Logical Operator2/1
  Logical Operator2/1 -> FltStat/1
  Data Store Read1/1 -> Relational Operator/1
  Merge/1 -> Data Store Write2/1, Logical Operator2/2
  Data Store Read2/1 -> HoldPrevFltPath/1(In1)

== system SF015A_WhlImbRejctn/WhlImbRejctn/WhlImbRejctnPer1/WIR Diagnostics/FrequencyDiag ==
  WIRCmd : Inport
  FreqEst : Inport  Port=2
  Enable : Inport  Port=3
  CmdAmp : Inport  Port=4
  Constant1 : Constant  Value=0  OutDataTypeStr=boolean
  Constant13 : Constant  Value=0  OutDataTypeStr=boolean
  Constant2 : Constant  OutDataTypeStr=boolean
  Constant5 : Constant  Value=WhlImbRejctnFrqDiagcEna
  CopyRight2 : Subsystem  Description=|  mask(Copyright Information){none=on}
      | Copyright info block.                                               
      |                                                                     
      | Place copyright information at the top of every subsystem in design.
      mask prompts: none "No parameters"
      mask help: Place copyright information at the top of every subsystem in design.
      mask Display:
      | NxtrConf = 'Nexteer Confidential';
      | 
      | sys = bdroot; %handle for the current model ("system")
      | first = get_param(sys,'Created');
      | first = first(end-3:end);  %year is last four digits
      | 
      | last = get_param(sys,'LastModifiedDate');
      | if isempty(last)
      |     last = datestr(now,'yyyy');
      | else
      |     last = last(end-3:end);
      | end
      | 
      | if strcmp(first,last)
      |     fprintf('%s -- Copyright %s Nexteer',NxtrConf,first)
      | else
      |     fprintf('%s -- %s%s- %s Nexteer',NxtrConf,char(169),first,last)
      | end
  Data Store Read1 : DataStoreRead  Priority=1  DataStoreName=FrqDiagcFltFaild
      settings: AttributesFormatString=Priority:%<Priority>
  Data Store Read2 : DataStoreRead  DataStoreName=FrqDiagcFltRcvry  DataStoreElements=FrqDiagcFltRcvry.Sts
  Data Store Read4 : DataStoreRead  Priority=1  DataStoreName=FrqDiagcFltRst
      settings: AttributesFormatString=Priority:%<Priority>
  Data Store Write2 : DataStoreWrite  Priority=2  DataStoreName=FrqDiagcFltFaild
      settings: AttributesFormatString=Priority:%<Priority>
  Data Type Conversion : DataTypeConversion  OutDataTypeStr=boolean
  Data Type Conversion1 : DataTypeConversion  OutDataTypeStr=boolean
  EnableDiag : Subsystem  RequirementInfo={} %GIDa_e70893fa_b476_41fc_83f3_cd56d2261539  TreatAsAtomicUnit=on
  Enumerated Constant1 : simulink/Sources/Enumerated Constant  OutDataTypeStr=Enum: SigQlfr1  Value=SigQlfr1.SIGQLFR_FAILD  SampleTime=inf
  Fault_RcvryPath : Subsystem  TreatAsAtomicUnit=on
  FreqDiagFault : Subsystem  RequirementInfo={} %GIDa_823acb2c_63d2_4f8b_8737_5bdfc9749030  TreatAsAtomicUnit=on
  If : If  IfExpression=u1
  If1 : If  RequirementInfo={} %GIDa_84d76f80_37f5_41d4_ac0a_c93962678a05  IfExpression=u1
  If5 : If  RequirementInfo={} %GIDa_329d3e5e_6fe7_4407_98ef_92a7d72cbf0a  IfExpression=u1
  Logical Operator2 : Logic  Operator=OR  AllPortsSameDT=off  OutDataTypeStr=boolean
  Merge : Merge
  Merge1 : Merge
  Merge5 : Merge
  NoDiag : Subsystem  RequirementInfo={} %GIDa_2b829a4a_b804_4dfa_be7f_b9930fa6303f  TreatAsAtomicUnit=on
  NoFault : Subsystem  RequirementInfo={} %GIDa_4cd1cae6_1247_413b_bca5_d0a1fdb2931d  TreatAsAtomicUnit=on
  NoFaultPath : Subsystem  TreatAsAtomicUnit=on
  Relational Operator : RelationalOperator  Operator===  OutDataTypeStr=boolean
  FltStat : Outport
  wires:
  WIRCmd/1 -> EnableDiag/3(WIRCmd)
  FreqEst/1 -> EnableDiag/2(FreqEst)
  Enable/1 -> EnableDiag/4(Enable)
  Constant5/1 -> If1/1
  Merge1/1 -> If5/1
  CmdAmp/1 -> EnableDiag/1(WIRCmdAmp)
  If5/1 -> FreqDiagFault/Action
  If5/2 -> NoFault/Action
  FreqDiagFault/1(Output) -> Merge5/1
  NoFault/1(Output) -> Merge5/2
  Constant2/1 -> Data Type Conversion/1
  Constant13/1 -> Data Type Conversion1/1
  If1/1 -> EnableDiag/Action
  If1/2 -> NoDiag/Action
  EnableDiag/1(Output) -> Merge1/1
  NoDiag/1(Output) -> Merge1/2
  Constant1/1 -> NoDiag/1(Input)
  Data Type Conversion/1 -> FreqDiagFault/1(Input)
  Data Type Conversion1/1 -> NoFault/1(Input)
  Merge5/1 -> If/1
  Data Store Read4/1 -> Fault_RcvryPath/1(FltReset)
  If/1 -> Fault_RcvryPath/Action
  Fault_RcvryPath/1(FltFailed) -> Merge/1
  NoFaultPath/1(FltFailed) -> Merge/2
  If/2 -> NoFaultPath/Action
  Enumerated Constant1/1 -> Relational Operator/2
  Relational Operator/1 -> Logical Operator2/1
  Logical Operator2/1 -> FltStat/1
  Data Store Read2/1 -> Relational Operator/1
  Merge/1 -> Data Store Write2/1, Logical Operator2/2
  Data Store Read1/1 -> NoFaultPath/1(In1)

== system SF015A_WhlImbRejctn/WhlImbRejctn/WhlImbRejctnPer1/WIR Diagnostics/MaxMagDiag ==
  CmdAmp : Inport
  CopyRight2 : Subsystem  Description=|  mask(Copyright Information){none=on}
      | Copyright info block.                                               
      |                                                                     
      | Place copyright information at the top of every subsystem in design.
      mask prompts: none "No parameters"
      mask help: Place copyright information at the top of every subsystem in design.
      mask Display:
      | NxtrConf = 'Nexteer Confidential';
      | 
      | sys = bdroot; %handle for the current model ("system")
      | first = get_param(sys,'Created');
      | first = first(end-3:end);  %year is last four digits
      | 
      | last = get_param(sys,'LastModifiedDate');
      | if isempty(last)
      |     last = datestr(now,'yyyy');
      | else
      |     last = last(end-3:end);
      | end
      | 
      | if strcmp(first,last)
      |     fprintf('%s -- Copyright %s Nexteer',NxtrConf,first)
      | else
      |     fprintf('%s -- %s%s- %s Nexteer',NxtrConf,char(169),first,last)
      | end
  Data Store Read : DataStoreRead  DataStoreName=MaxMgnFltRcvry  DataStoreElements=MaxMgnFltRcvry.Sts
  Data Store Read1 : DataStoreRead  Priority=1  DataStoreName=MaxMgnFltFaild
      settings: AttributesFormatString=Priority:%<Priority>
  Data Store Read4 : DataStoreRead  Priority=1  DataStoreName=MaxMgnFltRst
      settings: AttributesFormatString=Priority:%<Priority>
  Data Store Write2 : DataStoreWrite  Priority=2  DataStoreName=MaxMgnFltFaild
      settings: AttributesFormatString=Priority:%<Priority>
  Enumerated Constant1 : simulink/Sources/Enumerated Constant  OutDataTypeStr=Enum: SigQlfr1  Value=SigQlfr1.SIGQLFR_FAILD  SampleTime=inf
  Fault_RcvryPath : Subsystem  TreatAsAtomicUnit=on
  HoldprevFltPath : Subsystem  TreatAsAtomicUnit=on
  If : If  IfExpression=u1
  Logical Operator2 : Logic  Operator=OR  AllPortsSameDT=off  OutDataTypeStr=boolean
  Magnitude Comparison : Subsystem
  Merge : Merge
  Relational Operator : RelationalOperator  Operator===  OutDataTypeStr=boolean
  FltStat : Outport
  wires:
  CmdAmp/1 -> Magnitude Comparison/1(WIRCmdAmp1)
  Data Store Read4/1 -> Fault_RcvryPath/1(FltReset)
  If/1 -> Fault_RcvryPath/Action
  Fault_RcvryPath/1(FltFailed) -> Merge/1
  HoldprevFltPath/1(FltFailed) -> Merge/2
  If/2 -> HoldprevFltPath/Action
  Data Store Read/1 -> Relational Operator/1
  Enumerated Constant1/1 -> Relational Operator/2
  Relational Operator/1 -> Logical Operator2/1
  Logical Operator2/1 -> FltStat/1
  Magnitude Comparison/1(MagDiag) -> If/1
  Data Store Read1/1 -> HoldprevFltPath/1(In1)
  Merge/1 -> Data Store Write2/1, Logical Operator2/2

== system SF015A_WhlImbRejctn/WhlImbRejctn/WhlImbRejctnPer1/WIR Diagnostics/Set NTC Block ==
  note: Logic for setting of NTC bit based on WheelFrequencyValid
      | signal has been removed.
  MaxMag : Inport
  DC Trend : Inport  Port=2
  FrqDiagc : Inport  Port=3
  WhlSpdCorrln : Inport  Port=4
  MaxPersis : Inport  Port=5
  Action Port : ActionPort  ActionType=then
  Bitwise Operator : simulink/Logic and Bit Operations/Bitwise Operator  logicop=OR  UseBitMask=off  NumInputPorts=5  BitMask=bin2dec('11011001')  BitMaskRealWorld=Stored Integer
  Constant11 : Constant  Value=NODEBSTEP_CNT_U16
  Constant4 : Constant  Value=WhlImbRejctnFltNtc
  CopyRight2 : Subsystem  Description=|  mask(Copyright Information){none=on}
      | Copyright info block.                                               
      |                                                                     
      | Place copyright information at the top of every subsystem in design.
      mask prompts: none "No parameters"
      mask help: Place copyright information at the top of every subsystem in design.
      mask Display:
      | NxtrConf = 'Nexteer Confidential';
      | 
      | sys = bdroot; %handle for the current model ("system")
      | first = get_param(sys,'Created');
      | first = first(end-3:end);  %year is last four digits
      | 
      | last = get_param(sys,'LastModifiedDate');
      | if isempty(last)
      |     last = datestr(now,'yyyy');
      | else
      |     last = last(end-3:end);
      | end
      | 
      | if strcmp(first,last)
      |     fprintf('%s -- Copyright %s Nexteer',NxtrConf,first)
      | else
      |     fprintf('%s -- %s%s- %s Nexteer',NxtrConf,char(169),first,last)
      | end
  Enumerated Constant10 : simulink/Sources/Enumerated Constant  OutDataTypeStr=Enum: NtcSts1  Value=NtcSts1.NTCSTS_FAILD  SampleTime=inf
  NTC Bit parameter info : Subsystem
  NTC Bit parameter info2 : Subsystem
  NTC Bit parameter info3 : Subsystem
  NTC Bit parameter info4 : Subsystem
  NTC Bit parameter info5 : Subsystem
  SetNtcSts_Wo_Trigger : Subsystem  mask(SetNTC_WOT){}
      mask help: SetNTC library block
  wires:
  DC Trend/1 -> NTC Bit parameter info2/1(Flag)
  FrqDiagc/1 -> NTC Bit parameter info3/1(Flag)
  WhlSpdCorrln/1 -> NTC Bit parameter info4/1(Flag)
  Bitwise Operator/1 -> SetNtcSts_Wo_Trigger/2(NtcStInfo)
  Enumerated Constant10/1 -> SetNtcSts_Wo_Trigger/3(NtcSts)
  Constant11/1 -> SetNtcSts_Wo_Trigger/4(DebStep)
  MaxMag/1 -> NTC Bit parameter info/1(Flag)
  NTC Bit parameter info/1(FltBit) -> Bitwise Operator/1
  MaxPersis/1 -> NTC Bit parameter info5/1(Flag)
  NTC Bit parameter info2/1(FltBit) -> Bitwise Operator/2
  NTC Bit parameter info3/1(FltBit) -> Bitwise Operator/3
  NTC Bit parameter info4/1(FltBit) -> Bitwise Operator/4
  NTC Bit parameter info5/1(FltBit) -> Bitwise Operator/5
  Constant4/1 -> SetNtcSts_Wo_Trigger/1(NtcNr)

== system SF015A_WhlImbRejctn/WhlImbRejctn/WhlImbRejctnPer1/WIR Diagnostics/Set NTC Block1 ==
  Action Port : ActionPort  ActionType=else
  Constant11 : Constant  Value=NODEBSTEP_CNT_U16
  Constant4 : Constant  Value=WhlImbRejctnFltNtc
  Constant5 : Constant  Value=0  OutDataTypeStr=uint8
  CopyRight2 : Subsystem  Description=|  mask(Copyright Information){none=on}
      | Copyright info block.                                               
      |                                                                     
      | Place copyright information at the top of every subsystem in design.
      mask prompts: none "No parameters"
      mask help: Place copyright information at the top of every subsystem in design.
      mask Display:
      | NxtrConf = 'Nexteer Confidential';
      | 
      | sys = bdroot; %handle for the current model ("system")
      | first = get_param(sys,'Created');
      | first = first(end-3:end);  %year is last four digits
      | 
      | last = get_param(sys,'LastModifiedDate');
      | if isempty(last)
      |     last = datestr(now,'yyyy');
      | else
      |     last = last(end-3:end);
      | end
      | 
      | if strcmp(first,last)
      |     fprintf('%s -- Copyright %s Nexteer',NxtrConf,first)
      | else
      |     fprintf('%s -- %s%s- %s Nexteer',NxtrConf,char(169),first,last)
      | end
  Enumerated Constant10 : simulink/Sources/Enumerated Constant  OutDataTypeStr=Enum: NtcSts1  Value=NtcSts1.NTCSTS_PASSD  SampleTime=inf
  SetNtcSts_Wo_Trigger : Subsystem  mask(SetNTC_WOT){}
      mask help: SetNTC library block
  wires:
  Enumerated Constant10/1 -> SetNtcSts_Wo_Trigger/3(NtcSts)
  Constant11/1 -> SetNtcSts_Wo_Trigger/4(DebStep)
  Constant4/1 -> SetNtcSts_Wo_Trigger/1(NtcNr)
  Constant5/1 -> SetNtcSts_Wo_Trigger/2(NtcStInfo)
